simulink model "PICalculation_ExampleV"  (Simulink 2.20)
settings: Solver=ode4  StartTime=0.0  StopTime=100  FixedStep=0.1  RelTol=1e-3  AbsTol=1e-6
libraries: DABLib x1
settings Model: ConsistencyChecking=off  RTWPlaceOutputsASAP=off

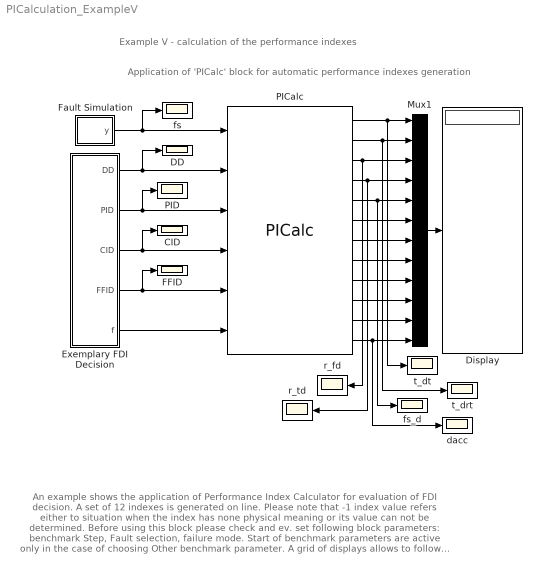
== system PICalculation_ExampleV ==
  note: Application of 'PICalc' block for automatic performance indexes generation
  note: Example V - calculation of the performance indexes
  note: An example shows the application of Performance Index
      | Calculator for evaluation of FDI decision. A set of  12 indexes is
      | generated on line. Please note that -1 index value refers either to
      | situation when the index has none physical meaning or its
      | value can not be determined. Before using this block please check
      | and ev. set following block parameters: benchmark Step, Fault
      |  selection, failure mode. Start of benchmark parameters are active only
      | in the case of choosing Other benchmark parameter. A grid of displays
      | allows to follow the  time evolution of performance indexes.  PICalc
      | must be supplied properly by the set of 6 input signals generated from FDI
      | system. The responsibility of creating the block interfacing PICalc
      |  lies on the FDI evaluator. For further details please refer to appropriate
      | section in Benchmark Definition description.
  CID : Scope
      settings: TickLabels=on  TimeRange=auto  YMin=0  YMax=5  SaveToWorkspace=off  SaveName=ScopeData  LimitMaxRows=off
  DD : Scope
      settings: TickLabels=on  TimeRange=100  YMin=0  YMax=1.1  SaveToWorkspace=off  SaveName=ScopeData  LimitMaxRows=off
  Display : Display
      settings: Format=short
  Exemplary FDI Decision : Subsystem
  FFID : Scope
      settings: TickLabels=on  TimeRange=auto  YMin=0  YMax=1.1  SaveToWorkspace=off  SaveName=ScopeData  LimitMaxRows=off
  Fault Simulation : Subsystem  mask(Fault generator){From=25, To=75, MFS=1, FDT=25, FSD=1}
      mask prompts: MFS "Max Fault Strength:"; FDT "Fault Development Time:"; FSD "Direction:"
      mask help:
      | Used for generation of abrupt and incipient standarised fault strength values.
      |
      | Parameters:
      | From - fault start time [s]
      | To - fault decay time [s]
      | Max Fault Strength - maximum fault strength value that will be reached during simulation [standarised range - 0 1]
      | Fault Development Time - after this time Max Fault Strength will be reached [s]
      | Direction - defines the sign of fault strength.
      mask init:
      | if FDT==0
      |  FDS = 99999999999999999999999999;
      | else
      |  FDS = MFS / FDT;
      | end
      | if To==inf
      |  To = 99999999999999999999999999;
      | end
      | if FSD >= 0
      | FSD=1;
      | else
      | FSD=-1;
      | end
      mask Help: web( [ 'file:///' which('DABLib.pdf')]);
      mask Display: disp('FGen')
  Mux1 : Mux  Inputs=12
  PICalc : DABLib/PICalc  Step=Other  FSel=NO FAULT  FType=Abrupt - Small  t_on_ini=0  t_hor_ini=100
  PID : Scope
      settings: TickLabels=on  TimeRange=auto  YMin=0  YMax=1.1  SaveToWorkspace=off  SaveName=ScopeData  LimitMaxRows=off
  dacc : Scope
      settings: TickLabels=on  TimeRange=100  YMin=0  YMax=1.1  SaveToWorkspace=off  SaveName=ScopeData  LimitMaxRows=off
  fs : Scope
      settings: TickLabels=on  TimeRange=auto  YMin=0  YMax=1.1  SaveToWorkspace=off  SaveName=ScopeData  LimitMaxRows=off
  fs_d : Scope
      settings: TickLabels=on  TimeRange=100  YMin=-1  YMax=1.1  SaveToWorkspace=off  SaveName=ScopeData  LimitMaxRows=off
  r_fd : Scope
      settings: TickLabels=on  TimeRange=100  YMin=-1  YMax=1.1  SaveToWorkspace=off  SaveName=ScopeData  LimitMaxRows=off
  r_td : Scope
      settings: TickLabels=on  TimeRange=100  YMin=-1  YMax=1.1  SaveToWorkspace=off  SaveName=ScopeData  LimitMaxRows=off
  t_drt : Scope
      settings: TickLabels=on  TimeRange=100  YMin=-5  YMax=30  SaveToWorkspace=off  SaveName=ScopeData  LimitMaxRows=off
  t_dt : Scope
      settings: TickLabels=on  TimeRange=100  YMin=-5  YMax=11  SaveToWorkspace=off  SaveName=ScopeData  LimitMaxRows=off
  wires:
  Exemplary FDI Decision/2(PID) -> PID/1, PICalc/3
  PICalc/6 -> Mux1/6
  PICalc/7 -> Mux1/7
  PICalc/8 -> Mux1/8
  PICalc/9 -> Mux1/9
  PICalc/1 -> Mux1/1, t_dt/1
  PICalc/2 -> Mux1/2, t_drt/1
  PICalc/3 -> Mux1/3, r_fd/1
  PICalc/4 -> Mux1/4, r_td/1
  PICalc/5 -> Mux1/5, fs_d/1
  PICalc/12 -> Mux1/12, dacc/1
  Fault Simulation/1(y) -> fs/1, PICalc/1
  Exemplary FDI Decision/5(f) -> PICalc/6
  Mux1/1 -> Display/1
  PICalc/10 -> Mux1/10
  PICalc/11 -> Mux1/11
  Exemplary FDI Decision/3(CID) -> PICalc/4, CID/1
  Exemplary FDI Decision/4(FFID) -> PICalc/5, FFID/1
  Exemplary FDI Decision/1(DD) -> PICalc/2, DD/1

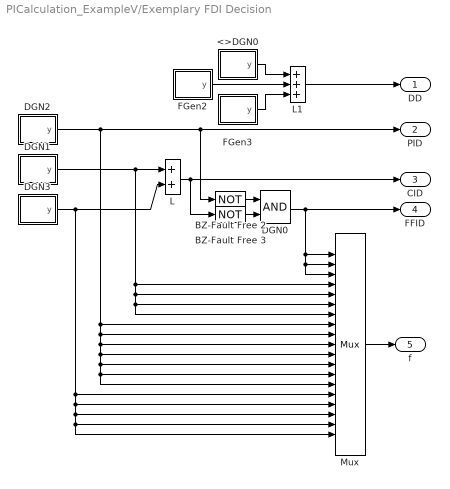
== system PICalculation_ExampleV/Exemplary FDI Decision ==
  <>DGN0 : Subsystem  mask(Fault generator){From=50, To=80, MFS=1, FDT=0, FSD=1}
      mask prompts: MFS "Max Fault Strength:"; FDT "Fault Development Time:"; FSD "Direction:"
      mask help:
      | Used for generation of abrupt and incipient standarised fault strength values.
      |
      | Parameters:
      | From - fault start time [s]
      | To - fault decay time [s]
      | Max Fault Strength - maximum fault strength value that will be reached during simulation [standarised range - 0 1]
      | Fault Development Time - after this time Max Fault Strength will be reached [s]
      | Direction - defines the sign of fault strength.
      mask init:
      | if FDT==0
      |  FDS = 99999999999999999999999999;
      | else
      |  FDS = MFS / FDT;
      | end
      | if To==inf
      |  To = 99999999999999999999999999;
      | end
      | if FSD >= 0
      | FSD=1;
      | else
      | FSD=-1;
      | end
      mask Help: web( [ 'file:///' which('DABLib.pdf')]);
      mask Display: disp('FGen')
  BZ-Fault Free 2 : Logic  Operator=NOT  Inputs=1
  BZ-Fault Free 3 : Logic  Operator=NOT  Inputs=1
  DGN0 : Logic  Operator=AND  Inputs=2
  DGN1 : Subsystem  mask(Fault generator){From=25, To=35, MFS=1, FDT=0, FSD=1}
      mask prompts: MFS "Max Fault Strength:"; FDT "Fault Development Time:"; FSD "Direction:"
      mask help:
      | Used for generation of abrupt and incipient standarised fault strength values.
      |
      | Parameters:
      | From - fault start time [s]
      | To - fault decay time [s]
      | Max Fault Strength - maximum fault strength value that will be reached during simulation [standarised range - 0 1]
      | Fault Development Time - after this time Max Fault Strength will be reached [s]
      | Direction - defines the sign of fault strength.
      mask init:
      | if FDT==0
      |  FDS = 99999999999999999999999999;
      | else
      |  FDS = MFS / FDT;
      | end
      | if To==inf
      |  To = 99999999999999999999999999;
      | end
      | if FSD >= 0
      | FSD=1;
      | else
      | FSD=-1;
      | end
      mask Help: web( [ 'file:///' which('DABLib.pdf')]);
      mask Display: disp('FGen')
  DGN2 : Subsystem  mask(Fault generator){From=45, To=50, MFS=1, FDT=0, FSD=1}
      mask prompts: MFS "Max Fault Strength:"; FDT "Fault Development Time:"; FSD "Direction:"
      mask help:
      | Used for generation of abrupt and incipient standarised fault strength values.
      |
      | Parameters:
      | From - fault start time [s]
      | To - fault decay time [s]
      | Max Fault Strength - maximum fault strength value that will be reached during simulation [standarised range - 0 1]
      | Fault Development Time - after this time Max Fault Strength will be reached [s]
      | Direction - defines the sign of fault strength.
      mask init:
      | if FDT==0
      |  FDS = 99999999999999999999999999;
      | else
      |  FDS = MFS / FDT;
      | end
      | if To==inf
      |  To = 99999999999999999999999999;
      | end
      | if FSD >= 0
      | FSD=1;
      | else
      | FSD=-1;
      | end
      mask Help: web( [ 'file:///' which('DABLib.pdf')]);
      mask Display: disp('FGen')
  DGN3 : Subsystem  mask(Fault generator){From=30, To=40, MFS=1, FDT=0, FSD=1}
      mask prompts: MFS "Max Fault Strength:"; FDT "Fault Development Time:"; FSD "Direction:"
      mask help:
      | Used for generation of abrupt and incipient standarised fault strength values.
      |
      | Parameters:
      | From - fault start time [s]
      | To - fault decay time [s]
      | Max Fault Strength - maximum fault strength value that will be reached during simulation [standarised range - 0 1]
      | Fault Development Time - after this time Max Fault Strength will be reached [s]
      | Direction - defines the sign of fault strength.
      mask init:
      | if FDT==0
      |  FDS = 99999999999999999999999999;
      | else
      |  FDS = MFS / FDT;
      | end
      | if To==inf
      |  To = 99999999999999999999999999;
      | end
      | if FSD >= 0
      | FSD=1;
      | else
      | FSD=-1;
      | end
      mask Help: web( [ 'file:///' which('DABLib.pdf')]);
      mask Display: disp('FGen')
  FGen2 : Subsystem  mask(Fault generator){From=35, To=45, MFS=1, FDT=0, FSD=1}
      mask prompts: MFS "Max Fault Strength:"; FDT "Fault Development Time:"; FSD "Direction:"
      mask help:
      | Used for generation of abrupt and incipient standarised fault strength values.
      |
      | Parameters:
      | From - fault start time [s]
      | To - fault decay time [s]
      | Max Fault Strength - maximum fault strength value that will be reached during simulation [standarised range - 0 1]
      | Fault Development Time - after this time Max Fault Strength will be reached [s]
      | Direction - defines the sign of fault strength.
      mask init:
      | if FDT==0
      |  FDS = 99999999999999999999999999;
      | else
      |  FDS = MFS / FDT;
      | end
      | if To==inf
      |  To = 99999999999999999999999999;
      | end
      | if FSD >= 0
      | FSD=1;
      | else
      | FSD=-1;
      | end
      mask Help: web( [ 'file:///' which('DABLib.pdf')]);
      mask Display: disp('FGen')
  FGen3 : Subsystem  mask(Fault generator){From=90, To=95, MFS=1, FDT=0, FSD=1}
      mask prompts: MFS "Max Fault Strength:"; FDT "Fault Development Time:"; FSD "Direction:"
      mask help:
      | Used for generation of abrupt and incipient standarised fault strength values.
      |
      | Parameters:
      | From - fault start time [s]
      | To - fault decay time [s]
      | Max Fault Strength - maximum fault strength value that will be reached during simulation [standarised range - 0 1]
      | Fault Development Time - after this time Max Fault Strength will be reached [s]
      | Direction - defines the sign of fault strength.
      mask init:
      | if FDT==0
      |  FDS = 99999999999999999999999999;
      | else
      |  FDS = MFS / FDT;
      | end
      | if To==inf
      |  To = 99999999999999999999999999;
      | end
      | if FSD >= 0
      | FSD=1;
      | else
      | FSD=-1;
      | end
      mask Help: web( [ 'file:///' which('DABLib.pdf')]);
      mask Display: disp('FGen')
  L : Sum  Inputs=++
  L1 : Sum  Inputs=+++
  Mux : Mux  Inputs=19
  DD : Outport  Port=1  InitialOutput=0
  PID : Outport  Port=2  InitialOutput=0
  CID : Outport  Port=3  InitialOutput=0
  FFID : Outport  Port=4  InitialOutput=0
  f : Outport  Port=5  InitialOutput=0
  wires:
  L/1 -> BZ-Fault Free 3/1, CID/1
  DGN0/1 -> Mux/1, Mux/2, Mux/3, FFID/1
  DGN1/1(y) -> L/1, Mux/4, Mux/5, Mux/6, Mux/7
  DGN2/1(y) -> BZ-Fault Free 2/1, PID/1, Mux/8, Mux/9, Mux/10, Mux/11, Mux/12, Mux/13, Mux/14
  DGN3/1(y) -> L/2, Mux/15, Mux/16, Mux/17, Mux/18, Mux/19
  Mux/1 -> f/1
  BZ-Fault Free 2/1 -> DGN0/1
  BZ-Fault Free 3/1 -> DGN0/2
  <>DGN0/1(y) -> L1/1
  FGen2/1(y) -> L1/2
  FGen3/1(y) -> L1/3
  L1/1 -> DD/1

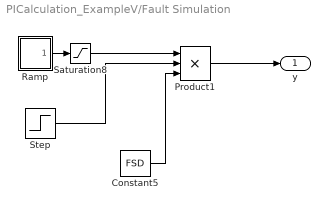
== system PICalculation_ExampleV/Fault Simulation ==
  Constant5 : Constant  Value=FSD
  Product1 : Product  Inputs=3
  Ramp : Subsystem  mask(Ramp){slope=FDS, start=From, X0=0}
      mask prompts: start "Start time:"; X0 "Initial output:"
      mask help: ramp
      mask Display: plot([0:10],[1,1,1,1:8])
  Saturation8 : Saturate  UpperLimit=MFS  LowerLimit=0
  Step : Step  Time=To  Before=1  After=0
  y : Outport  Port=1  InitialOutput=0
  wires:
  Ramp/1(out1) -> Saturation8/1
  Saturation8/1 -> Product1/1
  Step/1 -> Product1/2
  Product1/1 -> y/1
  Constant5/1 -> Product1/3

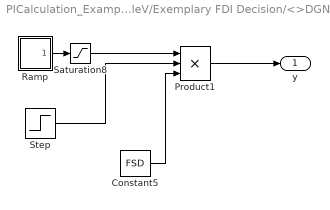
== system PICalculation_ExampleV/Exemplary FDI Decision/<>DGN0 ==
  Constant5 : Constant  Value=FSD
  Product1 : Product  Inputs=3
  Ramp : Subsystem  mask(Ramp){slope=FDS, start=From, X0=0}
      mask prompts: start "Start time:"; X0 "Initial output:"
      mask help: ramp
      mask Display: plot([0:10],[1,1,1,1:8])
  Saturation8 : Saturate  UpperLimit=MFS  LowerLimit=0
  Step : Step  Time=To  Before=1  After=0
  y : Outport  Port=1  InitialOutput=0
  wires:
  Ramp/1(out1) -> Saturation8/1
  Saturation8/1 -> Product1/1
  Step/1 -> Product1/2
  Product1/1 -> y/1
  Constant5/1 -> Product1/3

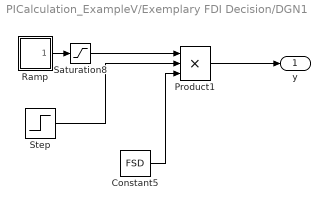
== system PICalculation_ExampleV/Exemplary FDI Decision/DGN1 ==
  Constant5 : Constant  Value=FSD
  Product1 : Product  Inputs=3
  Ramp : Subsystem  mask(Ramp){slope=FDS, start=From, X0=0}
      mask prompts: start "Start time:"; X0 "Initial output:"
      mask help: ramp
      mask Display: plot([0:10],[1,1,1,1:8])
  Saturation8 : Saturate  UpperLimit=MFS  LowerLimit=0
  Step : Step  Time=To  Before=1  After=0
  y : Outport  Port=1  InitialOutput=0
  wires:
  Ramp/1(out1) -> Saturation8/1
  Saturation8/1 -> Product1/1
  Step/1 -> Product1/2
  Product1/1 -> y/1
  Constant5/1 -> Product1/3

== system PICalculation_ExampleV/Exemplary FDI Decision/DGN2 ==
  Constant5 : Constant  Value=FSD
  Product1 : Product  Inputs=3
  Ramp : Subsystem  mask(Ramp){slope=FDS, start=From, X0=0}
      mask prompts: start "Start time:"; X0 "Initial output:"
      mask help: ramp
      mask Display: plot([0:10],[1,1,1,1:8])
  Saturation8 : Saturate  UpperLimit=MFS  LowerLimit=0
  Step : Step  Time=To  Before=1  After=0
  y : Outport  Port=1  InitialOutput=0
  wires:
  Ramp/1(out1) -> Saturation8/1
  Saturation8/1 -> Product1/1
  Step/1 -> Product1/2
  Product1/1 -> y/1
  Constant5/1 -> Product1/3

== system PICalculation_ExampleV/Exemplary FDI Decision/DGN3 ==
  Constant5 : Constant  Value=FSD
  Product1 : Product  Inputs=3
  Ramp : Subsystem  mask(Ramp){slope=FDS, start=From, X0=0}
      mask prompts: start "Start time:"; X0 "Initial output:"
      mask help: ramp
      mask Display: plot([0:10],[1,1,1,1:8])
  Saturation8 : Saturate  UpperLimit=MFS  LowerLimit=0
  Step : Step  Time=To  Before=1  After=0
  y : Outport  Port=1  InitialOutput=0
  wires:
  Ramp/1(out1) -> Saturation8/1
  Saturation8/1 -> Product1/1
  Step/1 -> Product1/2
  Product1/1 -> y/1
  Constant5/1 -> Product1/3

== system PICalculation_ExampleV/Exemplary FDI Decision/FGen2 ==
  Constant5 : Constant  Value=FSD
  Product1 : Product  Inputs=3
  Ramp : Subsystem  mask(Ramp){slope=FDS, start=From, X0=0}
      mask prompts: start "Start time:"; X0 "Initial output:"
      mask help: ramp
      mask Display: plot([0:10],[1,1,1,1:8])
  Saturation8 : Saturate  UpperLimit=MFS  LowerLimit=0
  Step : Step  Time=To  Before=1  After=0
  y : Outport  Port=1  InitialOutput=0
  wires:
  Ramp/1(out1) -> Saturation8/1
  Saturation8/1 -> Product1/1
  Step/1 -> Product1/2
  Product1/1 -> y/1
  Constant5/1 -> Product1/3

== system PICalculation_ExampleV/Exemplary FDI Decision/FGen3 ==
  Constant5 : Constant  Value=FSD
  Product1 : Product  Inputs=3
  Ramp : Subsystem  mask(Ramp){slope=FDS, start=From, X0=0}
      mask prompts: start "Start time:"; X0 "Initial output:"
      mask help: ramp
      mask Display: plot([0:10],[1,1,1,1:8])
  Saturation8 : Saturate  UpperLimit=MFS  LowerLimit=0
  Step : Step  Time=To  Before=1  After=0
  y : Outport  Port=1  InitialOutput=0
  wires:
  Ramp/1(out1) -> Saturation8/1
  Saturation8/1 -> Product1/1
  Step/1 -> Product1/2
  Product1/1 -> y/1
  Constant5/1 -> Product1/3

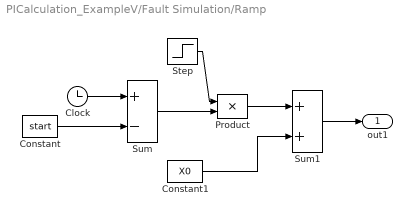
== system PICalculation_ExampleV/Fault Simulation/Ramp ==
  Clock : Clock
  Constant : Constant  Value=start
  Constant1 : Constant  Value=X0
  Product : Product  Inputs=2
  Step : Step  Time=start  Before=0  After=slope
  Sum : Sum  Inputs=+-
  Sum1 : Sum  Inputs=++
  out1 : Outport  Port=1
  wires:
  Sum/1 -> Product/2
  Constant/1 -> Sum/2
  Clock/1 -> Sum/1
  Step/1 -> Product/1
  Product/1 -> Sum1/1
  Constant1/1 -> Sum1/2
  Sum1/1 -> out1/1

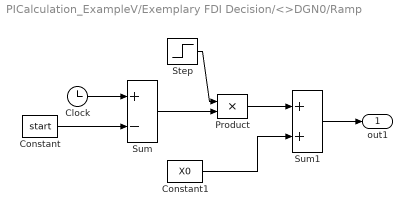
== system PICalculation_ExampleV/Exemplary FDI Decision/<>DGN0/Ramp ==
  Clock : Clock
  Constant : Constant  Value=start
  Constant1 : Constant  Value=X0
  Product : Product  Inputs=2
  Step : Step  Time=start  Before=0  After=slope
  Sum : Sum  Inputs=+-
  Sum1 : Sum  Inputs=++
  out1 : Outport  Port=1
  wires:
  Sum/1 -> Product/2
  Constant/1 -> Sum/2
  Clock/1 -> Sum/1
  Step/1 -> Product/1
  Product/1 -> Sum1/1
  Constant1/1 -> Sum1/2
  Sum1/1 -> out1/1

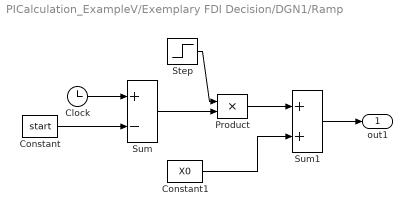
== system PICalculation_ExampleV/Exemplary FDI Decision/DGN1/Ramp ==
  Clock : Clock
  Constant : Constant  Value=start
  Constant1 : Constant  Value=X0
  Product : Product  Inputs=2
  Step : Step  Time=start  Before=0  After=slope
  Sum : Sum  Inputs=+-
  Sum1 : Sum  Inputs=++
  out1 : Outport  Port=1
  wires:
  Sum/1 -> Product/2
  Constant/1 -> Sum/2
  Clock/1 -> Sum/1
  Step/1 -> Product/1
  Product/1 -> Sum1/1
  Constant1/1 -> Sum1/2
  Sum1/1 -> out1/1

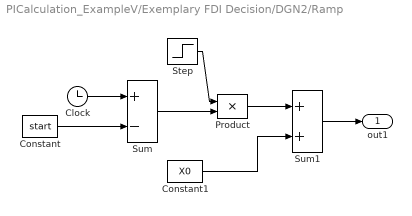
== system PICalculation_ExampleV/Exemplary FDI Decision/DGN2/Ramp ==
  Clock : Clock
  Constant : Constant  Value=start
  Constant1 : Constant  Value=X0
  Product : Product  Inputs=2
  Step : Step  Time=start  Before=0  After=slope
  Sum : Sum  Inputs=+-
  Sum1 : Sum  Inputs=++
  out1 : Outport  Port=1
  wires:
  Sum/1 -> Product/2
  Constant/1 -> Sum/2
  Clock/1 -> Sum/1
  Step/1 -> Product/1
  Product/1 -> Sum1/1
  Constant1/1 -> Sum1/2
  Sum1/1 -> out1/1

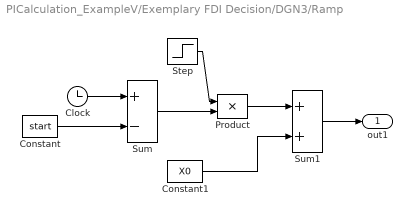
== system PICalculation_ExampleV/Exemplary FDI Decision/DGN3/Ramp ==
  Clock : Clock
  Constant : Constant  Value=start
  Constant1 : Constant  Value=X0
  Product : Product  Inputs=2
  Step : Step  Time=start  Before=0  After=slope
  Sum : Sum  Inputs=+-
  Sum1 : Sum  Inputs=++
  out1 : Outport  Port=1
  wires:
  Sum/1 -> Product/2
  Constant/1 -> Sum/2
  Clock/1 -> Sum/1
  Step/1 -> Product/1
  Product/1 -> Sum1/1
  Constant1/1 -> Sum1/2
  Sum1/1 -> out1/1

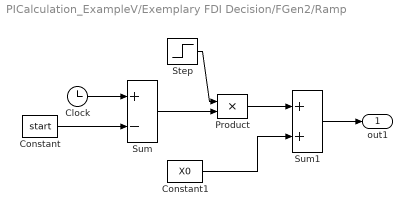
== system PICalculation_ExampleV/Exemplary FDI Decision/FGen2/Ramp ==
  Clock : Clock
  Constant : Constant  Value=start
  Constant1 : Constant  Value=X0
  Product : Product  Inputs=2
  Step : Step  Time=start  Before=0  After=slope
  Sum : Sum  Inputs=+-
  Sum1 : Sum  Inputs=++
  out1 : Outport  Port=1
  wires:
  Sum/1 -> Product/2
  Constant/1 -> Sum/2
  Clock/1 -> Sum/1
  Step/1 -> Product/1
  Product/1 -> Sum1/1
  Constant1/1 -> Sum1/2
  Sum1/1 -> out1/1

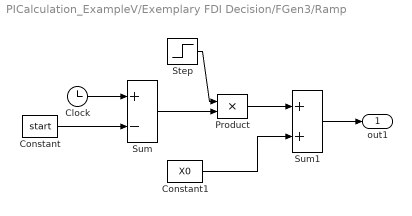
== system PICalculation_ExampleV/Exemplary FDI Decision/FGen3/Ramp ==
  Clock : Clock
  Constant : Constant  Value=start
  Constant1 : Constant  Value=X0
  Product : Product  Inputs=2
  Step : Step  Time=start  Before=0  After=slope
  Sum : Sum  Inputs=+-
  Sum1 : Sum  Inputs=++
  out1 : Outport  Port=1
  wires:
  Sum/1 -> Product/2
  Constant/1 -> Sum/2
  Clock/1 -> Sum/1
  Step/1 -> Product/1
  Product/1 -> Sum1/1
  Constant1/1 -> Sum1/2
  Sum1/1 -> out1/1
